simulink model "A450X"  (R2025b)
settings: Solver=ode23t  StartTime=0  StopTime=100  RelTol=1e-3
PreLoadFcn:
  | load terrain_data.mat
  | load NCM_TP_3700W_Pack.mat
undefined symbols (not defined in the file or in its folder): battery_builder_rtmsupport, gcbh
libraries: nesl_utility x34, fl_lib x21, NCM_TP_3700W_Pack_lib x15, sdl_lib x7, fl_ps_legacy_lib x2, ee_lib x1
(part 1 of 2)
settings Model: Creator=kanch  LastModifiedBy=kanch
settings DataIOCC: ExternalInput=[PedalTime,ThrottlePedal, FrontBrakePedal, RearBrakePedal]  LimitDataPoints=on  LoadExternalInput=on  SaveFormat=Array  DatasetSignalFormat=timetable

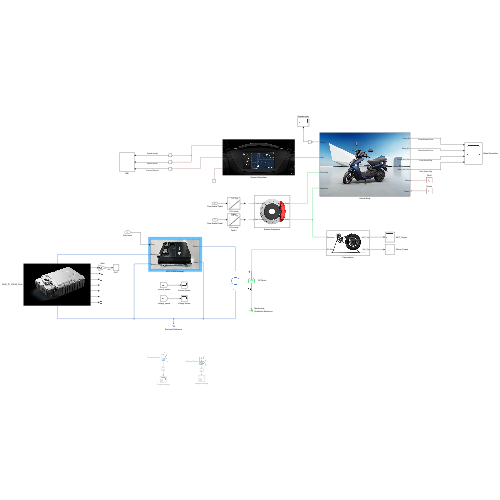
[thumbnail: Simulink's stored preview of the top-level diagram]
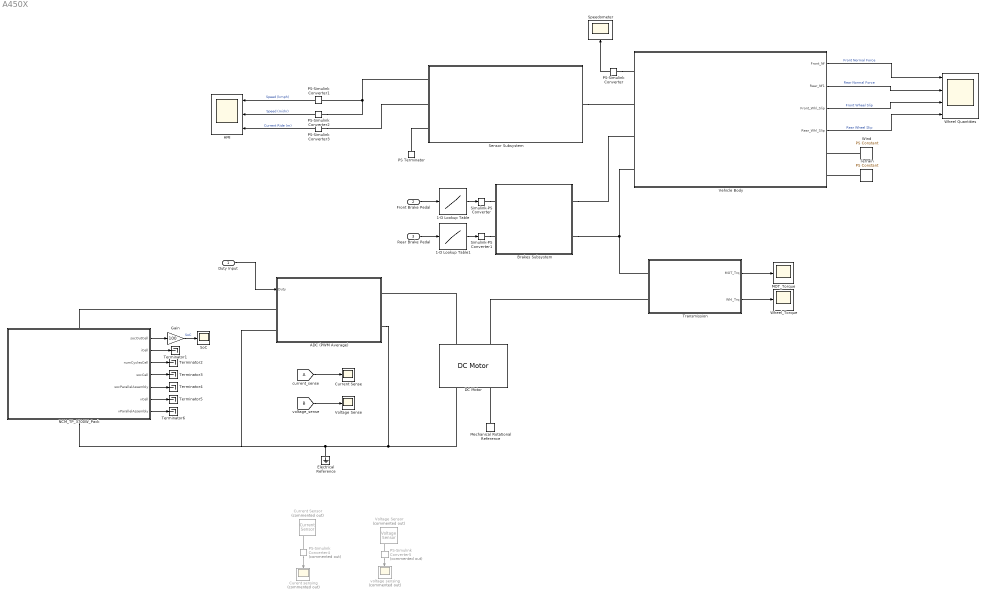
== system A450X ==
  Duty Input : Inport  OutDataTypeStr=double
  Front Brake Pedal : Inport  Port=2  OutDataTypeStr=double
  Rear Brake Pedal : Inport  Port=3  OutDataTypeStr=double
  1-D Lookup Table : Lookup_n-D  NumberOfTableDimensions=1  BreakpointsForDimension1=0:0.01:1  Table=0:10:1000  TableDataTypeStr=double  InternalRulePriority=Speed  RndMeth=Simplest
  1-D Lookup Table1 : Lookup_n-D  NumberOfTableDimensions=1  BreakpointsForDimension1=0:0.01:1  Table=0:10:1000  TableDataTypeStr=double  InternalRulePriority=Speed  RndMeth=Simplest
  ADC (PWM Average) : Subsystem
      mask Display: image('ADC.jpg');
  Brakes Subsystem : Subsystem
      mask Display: image('istockphoto-976970678-612x612.jpg');
  Curent sensing : Scope  Commented=on
      settings: ActiveDisplayYMinimum=-54.442210227956124  ActiveDisplayYMaximum=489.97989263859722  DataLoggingVariableName=ScopeData3
  Current Sense : Scope
      settings: ActiveDisplayYMinimum=-46.787986292582218  ActiveDisplayYMaximum=374.201526449331  DataLoggingVariableName=ScopeData5
  Current Sensor : fl_lib/Electrical/Electrical Sensors/Current Sensor  Commented=on
  DC Motor : ee_lib/Electromechanical/Brushed Motors/DC Motor  field_option=ee.enum.field_option.pm  Rf=100 Ohm  Lf=1 H  Laf=0.15 H  If0=0 A  parameterization=ee.enum.dcparam_option.load_speed  Ra=0.0093 Ohm  La=65 uH  emf_or_torque=2  Kv=0.19 V/(rad/s)  Ki=0.19 N*m/A  T_stall=2.4e-4 N*m  w_max=10000 rpm  w_rated=3000 rpm  P_rated=2.7 kW  V_rated=52 V  lam_param=1  i_noload=0 A  V_i_noload=1.5 V  J=0.001 kg*m^2  lam=1e-6 N*m/(rad/s)  speed0=0 rad/s  alpha=0.00393 1/K  Tmeas=25 C  thermal_mass=100 J/K  initial_temperature=25 C
  Electrical Reference : fl_lib/Electrical/Electrical Elements/Electrical Reference
  Gain : Gain  Gain=100
  HMI : Scope  NumInputPorts=3
      settings: ActiveDisplayYMinimum=-208.81866884061219  ActiveDisplayYMaximum=483.7407586284645
  MOT_Torque : Scope
      settings: ActiveDisplayYMinimum=-40.225007233877079  ActiveDisplayYMaximum=173.02081576612298
  Mechanical Rotational Reference : fl_lib/Mechanical/Rotational Elements/Mechanical Rotational Reference
  NCM_TP_3700W_Pack : Subsystem  LoadFcn=battery_builder_rtmsupport('loadfcn',gcbh);
      settings: CopyFcn=battery_builder_rtmsupport('copyfcn',gcbh);  PreCopyFcn=battery_builder_rtmsupport('precopyfcn',gcbh);  PreDeleteFcn=battery_builder_rtmsupport('predeletefcn',gcbh);  PortSchema="{\"entries\":[{\"content\":{\"sides\":[{\"content\":{\"connectorIds\":[\"LConn1\"]},\"type\":\"ConnectorPlacement.EquallySpacedRectSide\",\"uuid\":\"ade6cf47-5c74-4de5-b63e-38ab085eaa81\"},{\"content\":{\"connectorIds\":[\"RConn1\"],\"side\":\"RIGHT\"},\"type\":\"ConnectorPlacement.EquallySpacedRectSide\",\"uuid\":\"71e99cc0-4e29-44db-a862-89332aff9194\"},{\"content\":{\"side\":\"TOP\"},\"type\":\"ConnectorPlacement.EquallySpacedRectSide\",\"uuid\":\"ba61e147-4a7c-4984-85d5-ef017d8de781\"},{\"content\":{\"connectorIds\":[\"Out1\",\"Out2\",\"Out3\",\"Out4\",\"Out5\",\"Out6\",\"Out7\"],\"side\":\"BOTTOM\"},\"type\":\"ConnectorPlacement.EquallySpacedRectSide\",\"uuid\":\"7946668e-51c3-40d7-94f1-917450bfcc98\"}]},\"type\":\"ConnectorPlacement.EquallySpacedConnector\",\"uuid\":\"7b4d13cb-baf6-4c20-8350-11ac1ce882b9\"}],\"packageUris\":[\"http://schema.mathworks.com/mf0/Connector/R2020b\"],\"version\":\"1.0\"}"
      mask Display: image('450x_batterypack.jpg');
  PS Terminator : fl_lib/Physical Signals/Sinks/PS Terminator
  PS-Simulink Converter : nesl_utility/PS-Simulink Converter  PhysicalDomain=network_engine_domain  SubClassName=ps_output  LeftPortType=input  RightPortType=output  PseudoPeriodic=off  Frequencies=[]  VectorFormat=inherit  Unit=m/s  AffineConversion=off
  PS-Simulink Converter1 : nesl_utility/PS-Simulink Converter  PhysicalDomain=network_engine_domain  SubClassName=ps_output  LeftPortType=input  RightPortType=output  PseudoPeriodic=off  Frequencies=[]  VectorFormat=inherit  Unit=km/hr  AffineConversion=off
  PS-Simulink Converter2 : nesl_utility/PS-Simulink Converter  PhysicalDomain=network_engine_domain  SubClassName=ps_output  LeftPortType=input  RightPortType=output  PseudoPeriodic=off  Frequencies=[]  VectorFormat=inherit  Unit=mi/hr  AffineConversion=off
  PS-Simulink Converter3 : nesl_utility/PS-Simulink Converter  PhysicalDomain=network_engine_domain  SubClassName=ps_output  LeftPortType=input  RightPortType=output  PseudoPeriodic=off  Frequencies=[]  VectorFormat=inherit  Unit=m  AffineConversion=off
  PS-Simulink Converter4 : nesl_utility/PS-Simulink Converter  Commented=on  PhysicalDomain=network_engine_domain  SubClassName=ps_output  LeftPortType=input  RightPortType=output  PseudoPeriodic=off  Frequencies=[]  VectorFormat=inherit  Unit=A  AffineConversion=off
  PS-Simulink Converter5 : nesl_utility/PS-Simulink Converter  Commented=on  PhysicalDomain=network_engine_domain  SubClassName=ps_output  LeftPortType=input  RightPortType=output  PseudoPeriodic=off  Frequencies=[]  VectorFormat=inherit  Unit=V  AffineConversion=off
  Sensor Subsystem : Subsystem
      mask Display: image('Ather-450-dash-Google-Map-Platform.png');
  Simulink-PS Converter : nesl_utility/Simulink-PS Converter  PhysicalDomain=network_engine_domain  SubClassName=ps_input  LeftPortType=input  RightPortType=output  PseudoPeriodic=off  Frequencies=[]  NoiseDistribution=none  NoiseParameters=[]  Unit=1  AffineConversion=off  FilteringAndDerivatives=provide  SimscapeFilterOrder=1  InputFilterTimeConstant=0.001  UdotUserProvided=0
  Simulink-PS Converter1 : nesl_utility/Simulink-PS Converter  PhysicalDomain=network_engine_domain  SubClassName=ps_input  LeftPortType=input  RightPortType=output  PseudoPeriodic=off  Frequencies=[]  NoiseDistribution=none  NoiseParameters=[]  Unit=1  AffineConversion=off  FilteringAndDerivatives=provide  SimscapeFilterOrder=1  InputFilterTimeConstant=0.001  UdotUserProvided=0
  SoC : Scope
      settings: ActiveDisplayYMinimum=98.697081700360457  ActiveDisplayYMaximum=100.27611844811085
  Speedometer : Scope
      settings: Title=Velocity  ActiveDisplayYMinimum=-6.0123850448511007  ActiveDisplayYMaximum=31.432136047519947
  Terminator{1..6} (6 alike) : Terminator
  Terrain : fl_lib/Physical Signals/Sources/PS Constant  constant=0
  Transmission : Subsystem
      mask Display: image('450x_transmission.png');
  Vehicle Body : Subsystem
      mask Display: image('2025-450x6777c2f384486.png');
  Voltage Sense : Scope
      settings: ActiveDisplayYMinimum=39.7746283777626  ActiveDisplayYMaximum=63.090949336108665  DataLoggingVariableName=ScopeData6
  Voltage Sensor : fl_lib/Electrical/Electrical Sensors/Voltage Sensor  Commented=on
  Wheel Quantities : Scope  NumInputPorts=4
      settings: ActiveDisplayYMinimum=-235.90579329873469  ActiveDisplayYMaximum=1418.1170975012665  DataLoggingVariableName=ScopeData2
  Wheel_Torque : Scope
      settings: ActiveDisplayYMinimum=-36.602050520975681  ActiveDisplayYMaximum=187.30606362902427  DataLoggingVariableName=ScopeData2
  Wind : fl_lib/Physical Signals/Sources/PS Constant  constant=0 m/s
  current_sense : From  TagVisibility=global
  voltage sensing : Scope  Commented=on
      settings: ActiveDisplayYMinimum=58.152347575953634  ActiveDisplayYMaximum=63.41862804647986  DataLoggingVariableName=ScopeData4
  wires:
  PS-Simulink Converter/1 -> Speedometer/1
  PS-Simulink Converter1/1 -> HMI/1  "Speed (kmph)"
  PS-Simulink Converter2/1 -> HMI/2  "Speed (mi/hr)"
  PS-Simulink Converter3/1 -> HMI/3  "Current Ride (m)"
  1-D Lookup Table1/1 -> Simulink-PS Converter1/1
  1-D Lookup Table/1 -> Simulink-PS Converter/1
  NCM_TP_3700W_Pack/1(socOutCell) -> Gain/1
  NCM_TP_3700W_Pack/7(vParallelAssembly) -> Terminator6/1
  NCM_TP_3700W_Pack/6(vCell) -> Terminator5/1
  NCM_TP_3700W_Pack/5(socParallelAssembly) -> Terminator4/1
  NCM_TP_3700W_Pack/4(socCell) -> Terminator3/1
  NCM_TP_3700W_Pack/3(numCyclesCell) -> Terminator2/1
  NCM_TP_3700W_Pack/2(iCell) -> Terminator1/1
  Transmission/1(MOT_Trq) -> MOT_Torque/1
  Transmission/2(Whl_Trq) -> Wheel_Torque/1
  Vehicle Body/2(Rear_Nf1) -> Wheel Quantities/2  "Rear Normal Force"
  Vehicle Body/1(Front_Nf) -> Wheel Quantities/1  "Front Normal Force"
  Vehicle Body/3(Front_Whl_Slip) -> Wheel Quantities/3  "Front Wheel Slip"
  Vehicle Body/4(Rear_Whl_Slip) -> Wheel Quantities/4  "Rear Wheel Slip"
  Gain/1 -> SoC/1  "SoC"
  PS-Simulink Converter4/1 -> Curent sensing/1
  PS-Simulink Converter5/1 -> voltage sensing/1
  current_sense/1 -> Current Sense/1
  [B] -> Voltage Sense/1
  Duty Input/1 -> ADC (PWM Average)/1(Duty)
  Front Brake Pedal/1 -> 1-D Lookup Table/1
  Rear Brake Pedal/1 -> 1-D Lookup Table1/1
  connections:
  Wind/RConn1 -- Vehicle Body/RConn1
  PS-Simulink Converter/LConn1 -- Vehicle Body/LConn1
  PS-Simulink Converter2/LConn1 -- Sensor Subsystem/LConn1 -- PS-Simulink Converter1/LConn1
  Sensor Subsystem/RConn1 -- Vehicle Body/LConn2
  PS-Simulink Converter3/LConn1 -- Sensor Subsystem/LConn2
  Sensor Subsystem/LConn3 -- PS Terminator/LConn1
  Simulink-PS Converter1/RConn1 -- Brakes Subsystem/LConn2
  Simulink-PS Converter/RConn1 -- Brakes Subsystem/LConn1
  Terrain/RConn1 -- Vehicle Body/RConn2
  Brakes Subsystem/RConn1 -- Vehicle Body/LConn3
  Brakes Subsystem/RConn2 -- Transmission/LConn1 -- Vehicle Body/LConn4
  Electrical Reference/LConn1 -- ADC (PWM Average)/LConn2 -- NCM_TP_3700W_Pack/RConn1 -- ADC (PWM Average)/RConn2 -- DC Motor/RConn1
  Mechanical Rotational Reference/LConn1 -- DC Motor/RConn2
  Transmission/LConn2 -- DC Motor/LConn2
  PS-Simulink Converter4/LConn1 -- Current Sensor/RConn1
  PS-Simulink Converter5/LConn1 -- Voltage Sensor/RConn1
  ADC (PWM Average)/LConn1 -- NCM_TP_3700W_Pack/LConn1
  DC Motor/LConn1 -- ADC (PWM Average)/RConn1

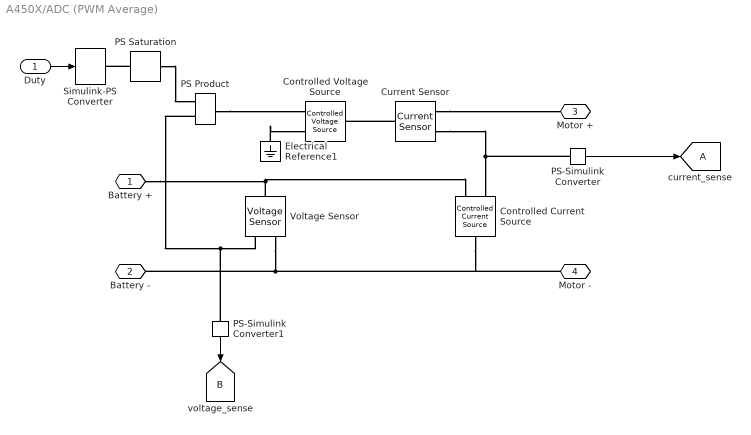
== system A450X/ADC (PWM Average) ==
  Duty : Inport
  Controlled Current Source : fl_lib/Electrical/Electrical Sources/Controlled Current Source
  Controlled Voltage Source : fl_lib/Electrical/Electrical Sources/Controlled Voltage Source
  Current Sensor : fl_lib/Electrical/Electrical Sensors/Current Sensor
  Electrical Reference1 : fl_lib/Electrical/Electrical Elements/Electrical Reference
  PS Product : fl_ps_legacy_lib/Legacy Physical Signals/Functions/PS Product
  PS Saturation : fl_ps_legacy_lib/Legacy Physical Signals/Nonlinear Operators/PS Saturation  upper_limit=1  lower_limit=0
      settings: InternalSimscapePortConfiguration="{\"Bottom\":[],\"Left\":[{\"id\":\"I\",\"label\":\"\",\"type\":\"input\"}],\"Right\":[{\"id\":\"O\",\"label\":\"\",\"type\":\"output\"}],\"Top\":[]}"
  PS-Simulink Converter : nesl_utility/PS-Simulink Converter  PhysicalDomain=network_engine_domain  SubClassName=ps_output  LeftPortType=input  RightPortType=output  PseudoPeriodic=off  Frequencies=[]  VectorFormat=inherit  Unit=inherit  AffineConversion=off
  PS-Simulink Converter1 : nesl_utility/PS-Simulink Converter  PhysicalDomain=network_engine_domain  SubClassName=ps_output  LeftPortType=input  RightPortType=output  PseudoPeriodic=off  Frequencies=[]  VectorFormat=inherit  Unit=inherit  AffineConversion=off
  Simulink-PS Converter : nesl_utility/Simulink-PS Converter  PhysicalDomain=network_engine_domain  SubClassName=ps_input  LeftPortType=input  RightPortType=output  PseudoPeriodic=off  Frequencies=[]  NoiseDistribution=none  NoiseParameters=[]  Unit=1  AffineConversion=off  FilteringAndDerivatives=zero  SimscapeFilterOrder=1  InputFilterTimeConstant=0.001  UdotUserProvided=1
  Voltage Sensor : fl_lib/Electrical/Electrical Sensors/Voltage Sensor
  current_sense : Goto  TagVisibility=global
  Battery + : PMIOPort  Side=Left
  Battery - : PMIOPort  Port=2  Side=Left
  Motor + : PMIOPort  Port=3  Side=Right
  Motor - : PMIOPort  Port=4  Side=Right
  tag scope: B=global
  wires:
  Duty/1 -> Simulink-PS Converter/1
  PS-Simulink Converter/1 -> current_sense/1
  PS-Simulink Converter1/1 -> [B]
  connections:
  Electrical Reference1/LConn1 -- Controlled Voltage Source/RConn2
  Current Sensor/LConn1 -- Controlled Voltage Source/LConn1
  Voltage Sensor/RConn2 -- Controlled Current Source/LConn1 -- Motor -/RConn1 -- Battery -/RConn1
  Current Sensor/RConn1 -- PS-Simulink Converter/LConn1 -- Controlled Current Source/RConn1
  PS Product/LConn2 -- PS-Simulink Converter1/LConn1 -- Voltage Sensor/RConn1
  Voltage Sensor/LConn1 -- Battery +/RConn1 -- Controlled Current Source/RConn2
  PS Product/RConn1 -- Controlled Voltage Source/RConn1
  Current Sensor/RConn2 -- Motor +/RConn1
  PS Saturation/RConn1 -- PS Product/LConn1
  PS Saturation/LConn1 -- Simulink-PS Converter/RConn1

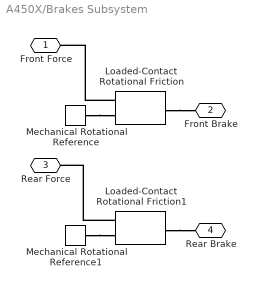
== system A450X/Brakes Subsystem ==
  Loaded-Contact Rotational Friction : sdl_lib/Brakes & Detents/Rotational/Loaded-Contact Rotational Friction  geometry_model=sdl.enum.friction_geometry.radius  r_eff=85 mm  d_o=150 mm  d_i=100 mm  friction_model=sdl.enum.friction_model_TLU_thermal.fixed  mu_w_vector=[0, 100, 1000] rad/s  temperature_TLU=[280, 300, 320] K  mu_static=0.35  mu_static_vector=[.4, .38, .36]  mu_coulomb=0.3  mu_coulomb_vector=[.3, .22, .19]  mu_coulomb_temp_vector=[.3, .28, .25]  mu_coulomb_matrix=[.34, .32, .3; .3, .28, .25; .25, .2, .15]  mu_interp_method=simscape.enum.interpolation.linear  mu_extrap_method=simscape.enum.extrapolation.linear  w_tol=0.001 rad/s  force_min=1 N  mu_visc=0 N*m*s/rad  initial_state_locked=sdl.enum.initial_lock.unlocked  thermal_mass=50 kJ/K  T_init=300 K
      settings: InternalSimscapePortConfiguration="{\"Bottom\":[],\"Left\":[{\"id\":\"N\",\"label\":\"N\",\"type\":\"input\"},{\"id\":\"B\",\"label\":\"B\",\"type\":\"foundation.mechanical.rotational.rotational\"}],\"Right\":[{\"id\":\"F\",\"label\":\"F\",\"type\":\"foundation.mechanical.rotational.rotational\"}],\"Top\":[]}"
  Loaded-Contact Rotational Friction1 : sdl_lib/Brakes & Detents/Rotational/Loaded-Contact Rotational Friction  geometry_model=sdl.enum.friction_geometry.radius  r_eff=80.75 mm  d_o=150 mm  d_i=100 mm  friction_model=sdl.enum.friction_model_TLU_thermal.fixed  mu_w_vector=[0, 100, 1000] rad/s  temperature_TLU=[280, 300, 320] K  mu_static=0.35  mu_static_vector=[.4, .38, .36]  mu_coulomb=0.3  mu_coulomb_vector=[.3, .22, .19]  mu_coulomb_temp_vector=[.3, .28, .25]  mu_coulomb_matrix=[.34, .32, .3; .3, .28, .25; .25, .2, .15]  mu_interp_method=simscape.enum.interpolation.linear  mu_extrap_method=simscape.enum.extrapolation.linear  w_tol=0.001 rad/s  force_min=1 N  mu_visc=0 N*m*s/rad  initial_state_locked=sdl.enum.initial_lock.unlocked  thermal_mass=50 kJ/K  T_init=300 K
      settings: InternalSimscapePortConfiguration="{\"Bottom\":[],\"Left\":[{\"id\":\"N\",\"label\":\"N\",\"type\":\"input\"},{\"id\":\"B\",\"label\":\"B\",\"type\":\"foundation.mechanical.rotational.rotational\"}],\"Right\":[{\"id\":\"F\",\"label\":\"F\",\"type\":\"foundation.mechanical.rotational.rotational\"}],\"Top\":[]}"
  Mechanical Rotational Reference : fl_lib/Mechanical/Rotational Elements/Mechanical Rotational Reference
  Mechanical Rotational Reference1 : fl_lib/Mechanical/Rotational Elements/Mechanical Rotational Reference
  Front Force : PMIOPort  Side=Left
  Front Brake : PMIOPort  Port=2  Side=Right
  Rear Force : PMIOPort  Port=3  Side=Left
  Rear Brake : PMIOPort  Port=4  Side=Right
  connections:
  Loaded-Contact Rotational Friction/RConn1 -- Front Brake/RConn1
  Mechanical Rotational Reference1/LConn1 -- Loaded-Contact Rotational Friction1/LConn2
  Loaded-Contact Rotational Friction1/LConn1 -- Rear Force/RConn1
  Mechanical Rotational Reference/LConn1 -- Loaded-Contact Rotational Friction/LConn2
  Loaded-Contact Rotational Friction/LConn1 -- Front Force/RConn1
  Loaded-Contact Rotational Friction1/RConn1 -- Rear Brake/RConn1

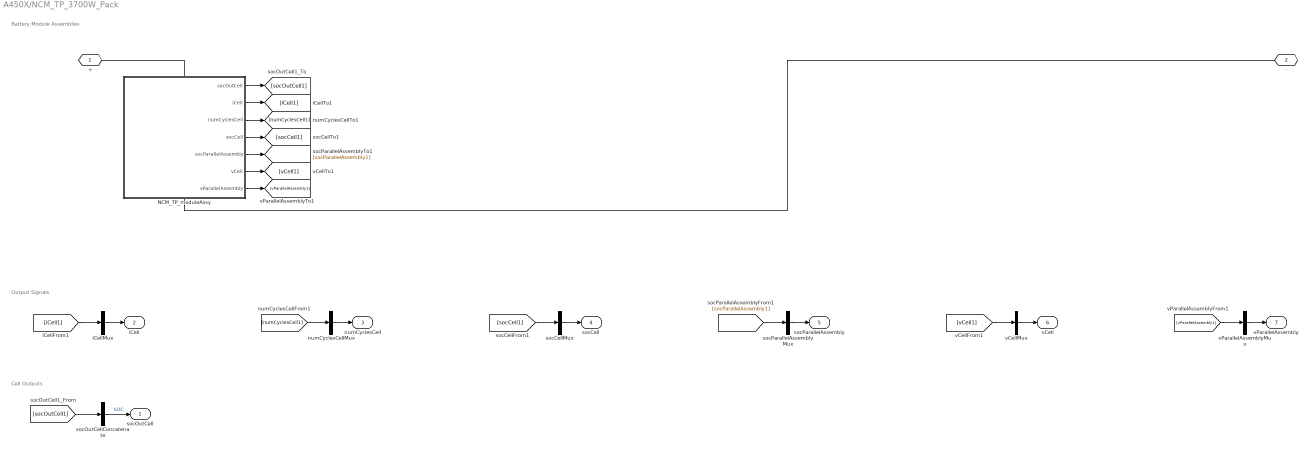
== system A450X/NCM_TP_3700W_Pack ==
  note: Battery Module Assemblies
  note: Output Signals
  note: Cell Outputs
  NCM_TP_moduleAssy : Subsystem  LoadFcn=battery_builder_rtmsupport('loadfcn',gcbh);
      settings: CopyFcn=battery_builder_rtmsupport('copyfcn',gcbh);  PreCopyFcn=battery_builder_rtmsupport('precopyfcn',gcbh);  PreDeleteFcn=battery_builder_rtmsupport('predeletefcn',gcbh);  PortSchema="{\"entries\":[{\"content\":{\"sides\":[{\"content\":{\"connectorIds\":[\"LConn1\"]},\"type\":\"ConnectorPlacement.EquallySpacedRectSide\",\"uuid\":\"ade6cf47-5c74-4de5-b63e-38ab085eaa81\"},{\"content\":{\"connectorIds\":[\"RConn1\"],\"side\":\"RIGHT\"},\"type\":\"ConnectorPlacement.EquallySpacedRectSide\",\"uuid\":\"71e99cc0-4e29-44db-a862-89332aff9194\"},{\"content\":{\"side\":\"TOP\"},\"type\":\"ConnectorPlacement.EquallySpacedRectSide\",\"uuid\":\"ba61e147-4a7c-4984-85d5-ef017d8de781\"},{\"content\":{\"connectorIds\":[\"Out1\",\"Out2\",\"Out3\",\"Out4\",\"Out5\",\"Out6\",\"Out7\"],\"side\":\"BOTTOM\"},\"type\":\"ConnectorPlacement.EquallySpacedRectSide\",\"uuid\":\"555fbbd9-b4bc-4141-9024-9c6d3292de07\"}]},\"type\":\"ConnectorPlacement.EquallySpacedConnector\",\"uuid\":\"7b4d13cb-baf6-4c20-8350-11ac1ce882b9\"}],\"packageUris\":[\"http://schema.mathworks.com/mf0/Connector/R2020b\"],\"version\":\"1.0\"}"
      mask Display: image('moduleAssembly_1.JPG');
  iCellMux : Mux  Inputs=1
  numCyclesCellMux : Mux  Inputs=1
  socCellMux : Mux  Inputs=1
  socOutCellConcatenate : Concatenate  NumInputs=1  Mode=Multidimensional array  ConcatenateDimension=2
  socParallelAssemblyMux : Mux  Inputs=1
  vCellMux : Mux  Inputs=1
  vParallelAssemblyMux : Mux  Inputs=1
  + : PMIOPort  Side=Left
  - : PMIOPort  Port=2  Side=Right
  socOutCell : Outport
  iCell : Outport  Port=2
  numCyclesCell : Outport  Port=3
  socCell : Outport  Port=4
  socParallelAssembly : Outport  Port=5
  vCell : Outport  Port=6
  vParallelAssembly : Outport  Port=7
  wires:
  socOutCellConcatenate/1 -> socOutCell/1  "SOC"
  [socOutCell1] -> socOutCellConcatenate/1
  NCM_TP_moduleAssy/2(iCell) -> [iCell1]
  iCellMux/1 -> iCell/1
  [iCell1] -> iCellMux/1
  NCM_TP_moduleAssy/3(numCyclesCell) -> [numCyclesCell1]
  numCyclesCellMux/1 -> numCyclesCell/1
  [numCyclesCell1] -> numCyclesCellMux/1
  NCM_TP_moduleAssy/4(socCell) -> [socCell1]
  socCellMux/1 -> socCell/1
  [socCell1] -> socCellMux/1
  NCM_TP_moduleAssy/5(socParallelAssembly) -> [socParallelAssembly1]
  socParallelAssemblyMux/1 -> socParallelAssembly/1
  [socParallelAssembly1] -> socParallelAssemblyMux/1
  NCM_TP_moduleAssy/6(vCell) -> [vCell1]
  vCellMux/1 -> vCell/1
  [vCell1] -> vCellMux/1
  NCM_TP_moduleAssy/7(vParallelAssembly) -> [vParallelAssembly1]
  vParallelAssemblyMux/1 -> vParallelAssembly/1
  [vParallelAssembly1] -> vParallelAssemblyMux/1
  NCM_TP_moduleAssy/1(socOutCell) -> [socOutCell1]
  connections:
  NCM_TP_moduleAssy/LConn1 -- +/RConn1
  NCM_TP_moduleAssy/RConn1 -- -/RConn1

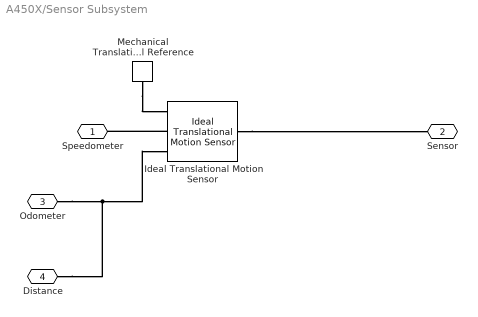
== system A450X/Sensor Subsystem ==
  Ideal Translational Motion Sensor : fl_lib/Mechanical/Mechanical Sensors/Ideal Translational Motion Sensor  reference=foundation.enum.MeasurementReference.difference  acceleration_port=false  velocity_port=true  position_port=true  offset=0 m
  Mechanical Translational Reference : fl_lib/Mechanical/Translational Elements/Mechanical Translational Reference
  Speedometer : PMIOPort  Side=Left
  Sensor : PMIOPort  Port=2  Side=Right
  Odometer : PMIOPort  Port=3  Side=Left
  Distance : PMIOPort  Port=4  Side=Left
  connections:
  Odometer/RConn1 -- Distance/RConn1 -- Ideal Translational Motion Sensor/RConn3
  Mechanical Translational Reference/LConn1 -- Ideal Translational Motion Sensor/RConn1
  Ideal Translational Motion Sensor/RConn2 -- Speedometer/RConn1
  Ideal Translational Motion Sensor/LConn1 -- Sensor/RConn1

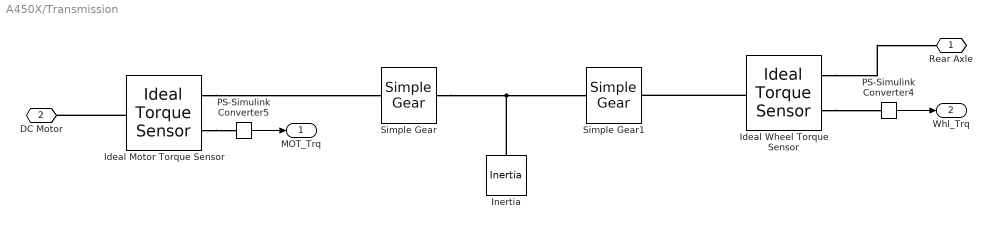
== system A450X/Transmission ==
  Ideal Motor Torque Sensor : fl_lib/Mechanical/Mechanical Sensors/Ideal Torque Sensor
  Ideal Wheel Torque Sensor : fl_lib/Mechanical/Mechanical Sensors/Ideal Torque Sensor
  Inertia : fl_lib/Mechanical/Rotational Elements/Inertia  inertia=0.01 kg*m^2  num_ports=foundation.enum.numPorts2.one  w_specify=off  w_priority=High  w=0 rad/s  w_nominal_specify=off  w_nominal_value=1  w_nominal_unit=rad/s  t_specify=off  t_priority=None  t=0 N*m  t_nominal_specify=off  t_nominal_value=1  t_nominal_unit=N*m
  PS-Simulink Converter4 : nesl_utility/PS-Simulink Converter  PhysicalDomain=network_engine_domain  SubClassName=ps_output  LeftPortType=input  RightPortType=output  PseudoPeriodic=off  Frequencies=[]  VectorFormat=inherit  Unit=N*m  AffineConversion=off
  PS-Simulink Converter5 : nesl_utility/PS-Simulink Converter  PhysicalDomain=network_engine_domain  SubClassName=ps_output  LeftPortType=input  RightPortType=output  PseudoPeriodic=off  Frequencies=[]  VectorFormat=inherit  Unit=N*m  AffineConversion=off
  Simple Gear : sdl_lib/Gears/Simple Gear  ratio=2.52  rotation_direction=sdl.enum.shaftOutputDirection.same  friction_model=sdl.enum.gear_efficiencies_load.off  T_noload=0.1 N*m  T_nom=5 N*m  efficiency_nom=0.8  efficiency=0.8  temperature_TLU=[280, 300, 320] K  load_TLU=[1, 5, 10] N*m  efficiency_TLU=[.95, .9, .85]  efficiency_TLU2=[.85, .8, .75; .95, .9, .85; .85, .8, .7]  w_thr=0.01 rad/s  pwr_thr=0.001 W  enable_backlash=false  hardstop_model=simscape.enum.hardstop.smooth  backlash_distance=1e-3 mm  r_base=0.1 m  transition=1e-4 mm  backlash_stiffness=1e6 N/m  backlash_damping=1e3 N*s/m  coeff_rest=0.7  v_tol=0.001 m/s  f_tol=0.001 N  mu_visc=[0, 0] N*m*s/rad  thermal_mass=50 J/K  temperature_specify=off  temperature_priority=High  temperature=300 K  temperature_nominal_specify=off  temperature_nominal_value=1  temperature_nominal_unit=K  x_backlash_specify=off  x_backlash_priority=None  x_backlash=0 mm  x_backlash_nominal_specify=off  x_backlash_nominal_value=1  x_backlash_nominal_unit=mm  f_hardstop_specify=off  f_hardstop_priority=None  f_hardstop=0 N  f_hardstop_nominal_specify=off  f_hardstop_nominal_value=1  f_hardstop_nominal_unit=N  v_backlash_specify=off  v_backlash_priority=None  v_backlash=0 m/s  v_backlash_nominal_specify=off  v_backlash_nominal_value=1  v_backlash_nominal_unit=m/s
  Simple Gear1 : sdl_lib/Gears/Simple Gear  ratio=3.09  rotation_direction=sdl.enum.shaftOutputDirection.same  friction_model=sdl.enum.gear_efficiencies_load.off  T_noload=0.1 N*m  T_nom=5 N*m  efficiency_nom=0.8  efficiency=0.8  temperature_TLU=[280, 300, 320] K  load_TLU=[1, 5, 10] N*m  efficiency_TLU=[.95, .9, .85]  efficiency_TLU2=[.85, .8, .75; .95, .9, .85; .85, .8, .7]  w_thr=0.01 rad/s  pwr_thr=0.001 W  enable_backlash=false  hardstop_model=simscape.enum.hardstop.smooth  backlash_distance=1e-3 mm  r_base=0.1 m  transition=1e-4 mm  backlash_stiffness=1e6 N/m  backlash_damping=1e3 N*s/m  coeff_rest=0.7  v_tol=0.001 m/s  f_tol=0.001 N  mu_visc=[0, 0] N*m*s/rad  thermal_mass=50 J/K  temperature_specify=off  temperature_priority=High  temperature=300 K  temperature_nominal_specify=off  temperature_nominal_value=1  temperature_nominal_unit=K  x_backlash_specify=off  x_backlash_priority=None  x_backlash=0 mm  x_backlash_nominal_specify=off  x_backlash_nominal_value=1  x_backlash_nominal_unit=mm  f_hardstop_specify=off  f_hardstop_priority=None  f_hardstop=0 N  f_hardstop_nominal_specify=off  f_hardstop_nominal_value=1  f_hardstop_nominal_unit=N  v_backlash_specify=off  v_backlash_priority=None  v_backlash=0 m/s  v_backlash_nominal_specify=off  v_backlash_nominal_value=1  v_backlash_nominal_unit=m/s
  Rear Axle : PMIOPort  Side=Left
  DC Motor : PMIOPort  Port=2  Side=Left
  MOT_Trq : Outport
  Whl_Trq : Outport  Port=2
  wires:
  PS-Simulink Converter4/1 -> Whl_Trq/1
  PS-Simulink Converter5/1 -> MOT_Trq/1
  connections:
  Ideal Motor Torque Sensor/LConn1 -- DC Motor/RConn1
  Ideal Wheel Torque Sensor/RConn2 -- PS-Simulink Converter4/LConn1
  Ideal Motor Torque Sensor/RConn2 -- PS-Simulink Converter5/LConn1
  Simple Gear/RConn1 -- Inertia/LConn1 -- Simple Gear1/LConn1
  Ideal Wheel Torque Sensor/LConn1 -- Simple Gear1/RConn1
  Ideal Motor Torque Sensor/RConn1 -- Simple Gear/LConn1
  Ideal Wheel Torque Sensor/RConn1 -- Rear Axle/RConn1

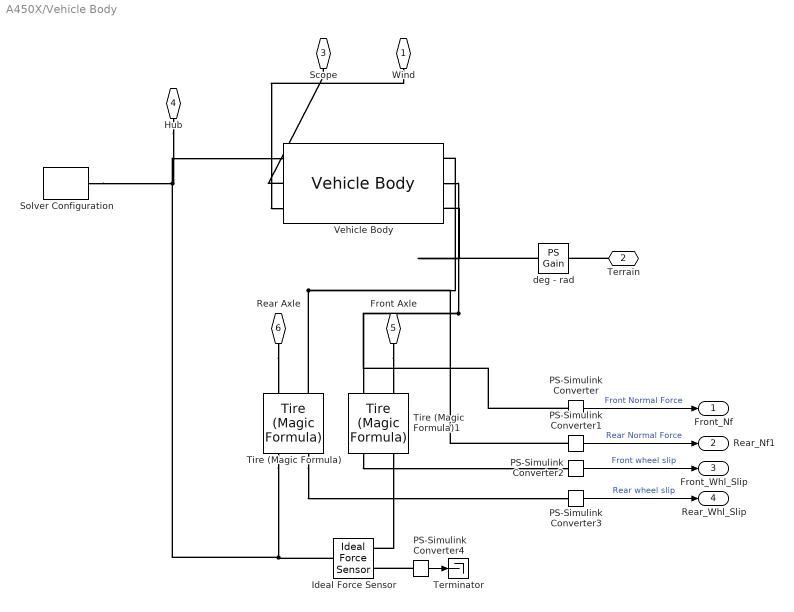
== system A450X/Vehicle Body ==
  Ideal Force Sensor : fl_lib/Mechanical/Mechanical Sensors/Ideal Force Sensor
  PS-Simulink Converter{,1..4} (5 alike) : nesl_utility/PS-Simulink Converter  PhysicalDomain=network_engine_domain  SubClassName=ps_output  LeftPortType=input  RightPortType=output  PseudoPeriodic=off  Frequencies=[]  VectorFormat=inherit  Unit=inherit  AffineConversion=off
  Solver Configuration : nesl_utility/Solver Configuration  PhysicalDomain=network_engine_domain  SubClassName=solver  LeftPortType=input  RightPortType=generic  Tones=[]  Harmonics=[]  SimulateNoise=off  Profile=off  UseLocalSampling=off  EnableSwitchedLinearOptims=on  FrequencyDomain=off  UseCCode=off  RelTol=0.001  AbsTol=0.001  MinStep=1e-09  ToWorkspace=off  RevertToSquareIcSolve=off  NumHomotopyIterations=100  PhasorMode=off  PhasorModeNumHarmonics=1  ConsistencySolver=NEWTON_XTOL_AFTER_FTOL  IndexReductionMethod=DerivativeReplacement  DoDC=off  ResidualTolerance=1e-09  ConsistencyTolSource=GLOBAL  ConsistencyAbsTol=0.001  ConsistencyRelTol=0.001  ConsistencyTolFactor=0.001  UseLocalSolver=off  LocalSolverChoice=NE_BACKWARD_EULER_ADVANCER  ResolveIndetEquations=on  FunctionEvalNumThread=1  LocalSolverSampleTime=0.001  DoFixedCost=off  MaxNonlinIter=3  MaxModeIter=2  ComputeImpulses=off  ImpulseIterations=2  LinearAlgebra=auto  LinearAlgebraNumThread=0  EquationFormulation=NE_TIME_EF  DelaysMemoryBudget=1024  AutomaticFiltering=on  FilteringTimeConstant=0.001  PartitionStorageMethod=AS_NEEDED  PartitionMemoryBudget=1024  PartitionMethod=ROBUST  MultibodyUseLocalSolver=off  MultibodyLocalSolverChoice=ODE1  MultibodyLocalSolverSampleTime=0.001
  Terminator : Terminator
  Tire (Magic Formula) : sdl_lib/Tires & Vehicles/Tire (Magic Formula)  parameterization=sdl.enum.magic_tire_model.constant  F_z1=1080 N  F_x1=3500 N  kappa1=10  B_m=10  C_m=1.9  D_m=1  E_m=0.97  fz0=4000 N  p_Cx=1.685  p_Dx=[1.21, -.037]  p_Ex=[.344, .095, -.02, 0]  p_Kx=[21.51, -.163, .245]  p_Hx=[-.002, .002]  p_Vx=[0, 0]  rolling_radius_model=sdl.enum.RollingRadiusParameterization.Constant  r_e=0.225 m  r_0=0.3 m  breff=8.39  dreff=0.26  freff=0.074  q_re0=0.99  q_v1=0.008  longvl=17 m/s  cz=5e5 N/m  model_resistance=true  resistance_model=sdl.enum.rollingResistanceParameterization.constant  coeff=0.007  p_tire=250e3 Pa  alpha=-0.003  beta=0.97  coeff_a=84e-4  coeff_b=6.2e-4 s/m  coeff_c=1.6e-4 s^2/m^2  p_tire0=240e3 Pa  fz0_resistance=4000 N  vH0=16 m/s  q_Sy=[.0082, 0, .0014, .001, 0, 0, 1.08, -.5]  v_thr=0.001 m/s  enable_scaling_coefficients=false  lfzO=1  lcx=1  lmux=1  lex=1  lkx=1  lhx=1  lvx=1  lmy=1  model_compliance=sdl.enum.compliance.off  stiffness=1e6 N/m  damping=1000 N*s/m  model_inertia=sdl.enum.model_inertia.on  inertia=0.001 kg*m^2  initial_velocity=0 rpm  vxlow=1 m/s  v_tr_thr=0.1 m/s  kpumin=-1.5  kpumax=1.5
  Tire (Magic Formula)1 : sdl_lib/Tires & Vehicles/Tire (Magic Formula)  parameterization=sdl.enum.magic_tire_model.constant  F_z1=1080 N  F_x1=3500 N  kappa1=10  B_m=10  C_m=1.9  D_m=1  E_m=0.97  fz0=4000 N  p_Cx=1.685  p_Dx=[1.21, -.037]  p_Ex=[.344, .095, -.02, 0]  p_Kx=[21.51, -.163, .245]  p_Hx=[-.002, .002]  p_Vx=[0, 0]  rolling_radius_model=sdl.enum.RollingRadiusParameterization.Constant  r_e=0.225 m  r_0=0.3 m  breff=8.39  dreff=0.26  freff=0.074  q_re0=0.99  q_v1=0.008  longvl=17 m/s  cz=5e5 N/m  model_resistance=true  resistance_model=sdl.enum.rollingResistanceParameterization.constant  coeff=0.007  p_tire=250e3 Pa  alpha=-0.003  beta=0.97  coeff_a=84e-4  coeff_b=6.2e-4 s/m  coeff_c=1.6e-4 s^2/m^2  p_tire0=240e3 Pa  fz0_resistance=4000 N  vH0=16 m/s  q_Sy=[.0082, 0, .0014, .001, 0, 0, 1.08, -.5]  v_thr=0.001 m/s  enable_scaling_coefficients=false  lfzO=1  lcx=1  lmux=1  lex=1  lkx=1  lhx=1  lvx=1  lmy=1  model_compliance=sdl.enum.compliance.off  stiffness=1e6 N/m  damping=1000 N*s/m  model_inertia=sdl.enum.model_inertia.on  inertia=0.001 kg*m^2  initial_velocity=0 rpm  vxlow=1 m/s  v_tr_thr=0.1 m/s  kpumin=-1.5  kpumax=1.5
  Vehicle Body : sdl_lib/Tires & Vehicles/Vehicle Body  mass=108+56 kg  n_w=1  x_f=0.696 m  x_r=0.6 m  y_c=0.3 m  mass_var=false  g=9.81 m/s^2  liftoff_warning=false  area=0.823 m^2  Cd_var=false  Cd=0.4  rho=1.18 kg/m^3  model_pitch=false  inertia=4000 kg*m^2  suspension_model=sdl.enum.linearTLU.linear  k_f=1e4 N/m  b_f=1e4 N*s/m  k_r=1e4 N/m  b_r=1e4 N*s/m  k_f_TLU=[-2000, -1000, 0, 1000, 2000] N  x_f_TLU=[-.4, -.2, 0, .2, .4] m  b_f_TLU=[-200, -100, 0, 100, 200] N  v_f_TLU=[-4, -2, 0, 2, 4] m/s  k_r_TLU=[-2000, -1000, 0, 1000, 2000] N  x_r_TLU=[-.4, -.2, 0, .2, .4] m  b_r_TLU=[-200, -100, 0, 100, 200] N  v_r_TLU=[-4, -2, 0, 2, 4] m/s  interp_method=simscape.enum.interpolation.linear  extrap_method=simscape.enum.extrapolation.linear  model_hardstop=false  upper_bound_f=.25 m  lower_bound_f=-.25 m  stop_k_f=1e6 N/m  stop_b_f=150 N*s/m  upper_bound_r=.25 m  lower_bound_r=-.25 m  stop_k_r=1e6 N/m  stop_b_r=150 N*s/m  initial_pitch=0 rad  initial_pitch_rate=0 rad/s  v_specify=on  v_priority=High  v=0 kph  v_nominal_specify=off  v_nominal_value=1  v_nominal_unit=m/s
      settings: InternalSimscapePortConfiguration="{\"Bottom\":[{\"id\":\"NR\",\"label\":\"NR\",\"type\":\"output\"},{\"id\":\"NF\",\"label\":\"NF\",\"type\":\"output\"},{\"id\":\"beta\",\"label\":\"beta\",\"type\":\"input\"}],\"Left\":[{\"id\":\"H\",\"label\":\"H\",\"type\":\"foundation.mechanical.translational.translational\"}],\"Right\":[],\"Top\":[{\"id\":\"V\",\"label\":\"V\",\"type\":\"output\"},{\"id\":\"wind\",\"label\":\"W\",\"type\":\"input\"}]}"
  deg - rad : fl_lib/Physical Signals/Functions/PS Gain  gain=pi/180
  Wind : PMIOPort  Side=Right
  Terrain : PMIOPort  Port=2  Side=Right
  Scope : PMIOPort  Port=3  Side=Left
  Hub : PMIOPort  Port=4  Side=Left
  Front Axle : PMIOPort  Port=5  Side=Left
  Rear Axle : PMIOPort  Port=6  Side=Left
  Front_Nf : Outport
  Rear_Nf1 : Outport  Port=2
  Front_Whl_Slip : Outport  Port=3
  Rear_Whl_Slip : Outport  Port=4
  wires:
  PS-Simulink Converter4/1 -> Terminator/1
  PS-Simulink Converter/1 -> Front_Nf/1  "Front Normal Force"
  PS-Simulink Converter1/1 -> Rear_Nf1/1  "Rear Normal Force"
  PS-Simulink Converter2/1 -> Front_Whl_Slip/1  "Front wheel slip"
  PS-Simulink Converter3/1 -> Rear_Whl_Slip/1  "Rear wheel slip"
  connections:
  Tire (Magic Formula)/RConn2 -- Ideal Force Sensor/LConn1 -- Hub/RConn1 -- Vehicle Body/LConn1 -- Solver Configuration/RConn1
  Tire (Magic Formula)/LConn1 -- PS-Simulink Converter1/LConn1 -- Vehicle Body/RConn1
  deg - rad/RConn1 -- Vehicle Body/RConn3
  Vehicle Body/RConn2 -- PS-Simulink Converter/LConn1 -- Tire (Magic Formula)1/LConn1
  Front Axle/RConn1 -- Tire (Magic Formula)1/LConn2
  Rear Axle/RConn1 -- Tire (Magic Formula)/LConn2
  Terrain/RConn1 -- deg - rad/LConn1
  Wind/RConn1 -- Vehicle Body/LConn3
  Vehicle Body/LConn2 -- Scope/RConn1
  Tire (Magic Formula)1/RConn1 -- PS-Simulink Converter2/LConn1
  Tire (Magic Formula)/RConn1 -- PS-Simulink Converter3/LConn1
  Tire (Magic Formula)1/RConn2 -- Ideal Force Sensor/RConn1
  PS-Simulink Converter4/LConn1 -- Ideal Force Sensor/RConn2
